simulink library "Driveline_Axle3_A23_A2Diff_A3Diff"  (R2025b)
settings: Solver=VariableStepAuto  StartTime=0.0  StopTime=10.0  RelTol=1e-3
undefined symbols (not defined in the file): Driveline
libraries: Driveshaft_Assembly x4, fl_lib x3, Differential_Systems x2, sdl_lib x2, Driveline_Axle2_A1_A1Diff x2, sm_lib x1
Description:
  | Component of Simscape Vehicle Templates Library
  | 
  | Copyright 2018-2025 The MathWorks, Inc.
settings Model: Creator=smiller  LastModifiedBy=smiller
settings SolverCC: AlgebraicLoopSolver=TrustRegion
settings DataIOCC: ReturnWorkspaceOutputs=off
settings OptimizationCC: ReuseModelBlockBuffer=off
settings DebuggingCC: UnconnectedInputMsg=warning  UnconnectedOutputMsg=warning  UnconnectedLineMsg=warning  ArithmeticOperatorsInVariantConditions=warning
settings ModelReferenceCC: EnableRefExpFcnMdlSchedulingChecks=on
settings SFSimCC: CustomCodeUndefinedFunction=UseInterfaceOnly
settings RTWCC: GPUComputeCapability=3.5  DLArmComputeVersion=19.05

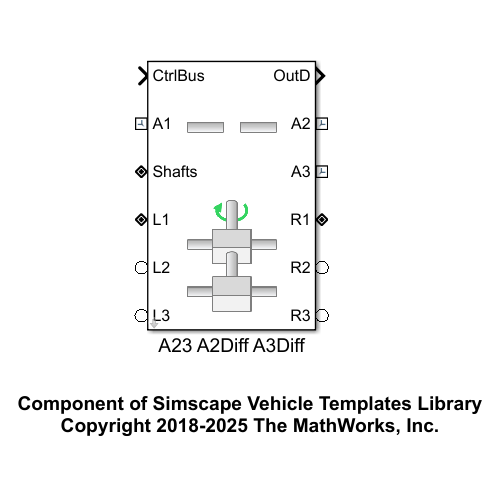
[thumbnail: Simulink's stored preview of the top-level diagram]
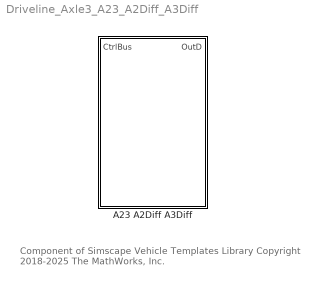
== system Driveline_Axle3_A23_A2Diff_A3Diff ==
  note: Component of Simscape Vehicle Templates Library
      | Copyright 2018-2025 The MathWorks, Inc.
  A23 A2Diff A3Diff : Subsystem  Tag=PublishSubsystem  VariantControl=IndepFRDiffFDiffR  mask(Driveline 6x4, 3-Axle, One Input Shaft){}
      mask help: Models driveline with 3 axles. The second and third axles are mechanically connected, and a single input shaft powers both axles.
      mask Display: image('sm_car_vehicle_driveline_axle3_a23_a2diff_a3diff_IMAGE.png');

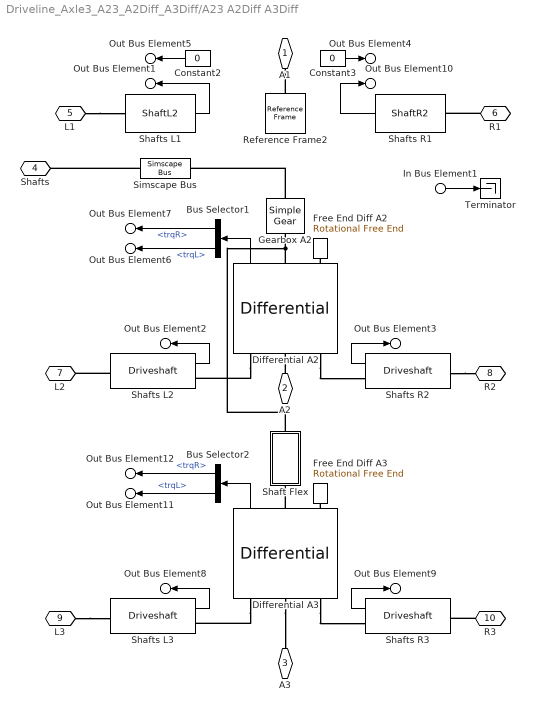
== system Driveline_Axle3_A23_A2Diff_A3Diff/A23 A2Diff A3Diff ==
  In Bus Element1 : Inport  PortName=CtrlBus
  Bus Selector1 : BusSelector  OutputSignals=trqR,trqL
  Bus Selector2 : BusSelector  OutputSignals=trqR,trqL
  Constant2 : Constant  Value=0
  Constant3 : Constant  Value=0
  Differential A2 : Differential_Systems/Differential  VariantControl=Variant1  LabelModeActiveChoice=Gear1DShafts1D  Differential=Driveline.DifferentialA2  VariantLabel=Driveline.DifferentialA2.class.Value
      settings: AttributesFormatString=%<ActiveVariant>
  Differential A3 : Differential_Systems/Differential  VariantControl=Variant1  LabelModeActiveChoice=Gear1DShafts1D  Differential=Driveline.DifferentialA3  VariantLabel=Driveline.DifferentialA3.class.Value
      settings: AttributesFormatString=%<ActiveVariant>
  Free End Diff A2 : fl_lib/Mechanical/Rotational Elements/Rotational Free End  w_specify=off  w_priority=None  w=0 rad/s  w_nominal_specify=off  w_nominal_value=1  w_nominal_unit=rad/s
  Free End Diff A3 : fl_lib/Mechanical/Rotational Elements/Rotational Free End  w_specify=off  w_priority=None  w=0 rad/s  w_nominal_specify=off  w_nominal_value=1  w_nominal_unit=rad/s
  Gearbox A2 : sdl_lib/Gears/Simple Gear  ratio=Driveline.GearboxA2.ratio.Value  rotation_direction=3-2*(1)  friction_model=1  T_noload=0.1 N*m  T_nom=5 N*m  efficiency_nom=0.8  efficiency=0.8  temperature_TLU=[280, 300, 320] K  load_TLU=[1, 5, 10] N*m  efficiency_TLU=[.95, .9, .85]  efficiency_TLU2=[.85, .8, .75; .95, .9, .85; .85, .8, .7]  w_thr=0.01 rad/s  pwr_thr=0.001 W  enable_backlash=false  hardstop_model=simscape.enum.hardstop.smooth  backlash_distance=1e-3 mm  r_base=0.1 m  transition=1e-4 mm  backlash_stiffness=1e7 N/m  backlash_damping=1e6 N*s/m  coeff_rest=0  v_tol=0.001 m/s  f_tol=0 N  mu_visc=[0, 0] N*m/(rad/s)  thermal_mass=50 J/K  temperature_specify=off  temperature_priority=High  temperature=300 K  temperature_nominal_specify=off  temperature_nominal_value=1  temperature_nominal_unit=K  x_backlash_specify=off  x_backlash_priority=None  x_backlash=0 mm  x_backlash_nominal_specify=off  x_backlash_nominal_value=1  x_backlash_nominal_unit=mm  f_hardstop_specify=off  f_hardstop_priority=None  f_hardstop=0 N  f_hardstop_nominal_specify=off  f_hardstop_nominal_value=1  f_hardstop_nominal_unit=N  v_backlash_specify=off  v_backlash_priority=None  v_backlash=0 m/s  v_backlash_nominal_specify=off  v_backlash_nominal_value=1  v_backlash_nominal_unit=m/s
  Reference Frame2 : sm_lib/Frames and Transforms/Reference Frame
  Shaft Flex : Subsystem
  Shafts L1 : Driveline_Axle2_A1_A1Diff/A1 A1Diff/ShaftL2  VariantControl=Shaft1D
  Shafts L2 : Driveshaft_Assembly/Driveshaft  VariantControl=Variant1  LabelModeActiveChoice=Shaft1D  popup_leftRight=Left  Driveshaft=Driveline.DriveshaftL2  VariantLabel=Driveline.DriveshaftL2.class.Value
      settings: AttributesFormatString=%<ActiveVariant>
  Shafts L3 : Driveshaft_Assembly/Driveshaft  VariantControl=Variant1  LabelModeActiveChoice=Shaft1D  popup_leftRight=Left  Driveshaft=Driveline.DriveshaftL3  VariantLabel=Driveline.DriveshaftL3.class.Value
      settings: AttributesFormatString=%<ActiveVariant>
  Shafts R1 : Driveline_Axle2_A1_A1Diff/A1 A1Diff/ShaftR2  VariantControl=Shaft1D
  Shafts R2 : Driveshaft_Assembly/Driveshaft  VariantControl=Variant1  LabelModeActiveChoice=Shaft1D  popup_leftRight=Right  Driveshaft=Driveline.DriveshaftR2  VariantLabel=Driveline.DriveshaftR2.class.Value
      settings: AttributesFormatString=%<ActiveVariant>
  Shafts R3 : Driveshaft_Assembly/Driveshaft  VariantControl=Variant1  LabelModeActiveChoice=Shaft1D  popup_leftRight=Right  Driveshaft=Driveline.DriveshaftR3  VariantLabel=Driveline.DriveshaftR3.class.Value
      settings: AttributesFormatString=%<ActiveVariant>
  Simscape Bus : SimscapeBus  HierarchyStrings=ShaftA2
  Terminator : Terminator
  A1 : PMIOPort  Side=Left
  A2 : PMIOPort  Port=2  Side=Right
  A3 : PMIOPort  Port=3  Side=Right
  Shafts : PMIOPort  Port=4  Side=Left
  L1 : PMIOPort  Port=5  Side=Left
  R1 : PMIOPort  Port=6  Side=Right
  L2 : PMIOPort  Port=7  Side=Left
  R2 : PMIOPort  Port=8  Side=Right
  L3 : PMIOPort  Port=9  Side=Left
  R3 : PMIOPort  Port=10  Side=Right
  Out Bus Element4 : Outport  VectorParamsAs1DForOutWhenUnconnected=off  PortName=OutD  Element=MDriveshaftR1
  Out Bus Element5 : Outport  VectorParamsAs1DForOutWhenUnconnected=off  PortName=OutD  Element=MDriveshaftL1
  Out Bus Element2 : Outport  VectorParamsAs1DForOutWhenUnconnected=off  PortName=OutD  Element=anDriveshaftL2
  Out Bus Element3 : Outport  VectorParamsAs1DForOutWhenUnconnected=off  PortName=OutD  Element=anDriveshaftR2
  Out Bus Element6 : Outport  VectorParamsAs1DForOutWhenUnconnected=off  PortName=OutD  Element=MDriveshaftL2
  Out Bus Element7 : Outport  VectorParamsAs1DForOutWhenUnconnected=off  PortName=OutD  Element=MDriveshaftR2
  Out Bus Element1 : Outport  VectorParamsAs1DForOutWhenUnconnected=off  PortName=OutD  Element=anDriveshaftL1
  Out Bus Element10 : Outport  VectorParamsAs1DForOutWhenUnconnected=off  PortName=OutD  Element=anDriveshaftR1
  Out Bus Element8 : Outport  VectorParamsAs1DForOutWhenUnconnected=off  PortName=OutD  Element=anDriveshaftL3
  Out Bus Element9 : Outport  VectorParamsAs1DForOutWhenUnconnected=off  PortName=OutD  Element=anDriveshaftR3
  Out Bus Element11 : Outport  VectorParamsAs1DForOutWhenUnconnected=off  PortName=OutD  Element=MDriveshaftL3
  Out Bus Element12 : Outport  VectorParamsAs1DForOutWhenUnconnected=off  PortName=OutD  Element=MDriveshaftR3
  wires:
  In Bus Element1/1 -> Terminator/1
  Shafts R2/1 -> Out Bus Element3/1
  Shafts L2/1 -> Out Bus Element2/1
  Differential A2/1 -> Bus Selector1/1
  Bus Selector1/1 -> Out Bus Element7/1  "<trqR>"
  Bus Selector1/2 -> Out Bus Element6/1  "<trqL>"
  Shafts L1/1 -> Out Bus Element1/1
  Shafts R1/1 -> Out Bus Element10/1
  Constant2/1 -> Out Bus Element5/1
  Constant3/1 -> Out Bus Element4/1
  Bus Selector2/2 -> Out Bus Element11/1  "<trqL>"
  Bus Selector2/1 -> Out Bus Element12/1  "<trqR>"
  Differential A3/1 -> Bus Selector2/1
  Shafts L3/1 -> Out Bus Element8/1
  Shafts R3/1 -> Out Bus Element9/1
  connections:
  Simscape Bus/RConn1 -- Shafts/RConn1
  Shafts L2/LConn1 -- L2/RConn1
  Shafts R2/LConn1 -- R2/RConn1
  R3/RConn1 -- Shafts R3/LConn1
  L3/RConn1 -- Shafts L3/LConn1
  A2/RConn1 -- Differential A2/LConn2
  Differential A2/LConn1 -- Shafts L2/RConn1
  Differential A2/LConn3 -- Shafts R2/RConn1
  Gearbox A2/LConn1 -- Simscape Bus/LConn1
  Differential A2/RConn2 -- Free End Diff A2/LConn1
  Differential A2/RConn1 -- Shaft Flex/LConn1 -- Gearbox A2/RConn1
  L1/RConn1 -- Shafts L1/LConn1
  R1/RConn1 -- Shafts R1/LConn1
  Reference Frame2/RConn1 -- A1/RConn1
  Differential A3/RConn2 -- Free End Diff A3/LConn1
  Differential A3/LConn3 -- Shafts R3/RConn1
  Differential A3/LConn1 -- Shafts L3/RConn1
  Differential A3/LConn2 -- A3/RConn1
  Differential A3/RConn1 -- Shaft Flex/RConn1

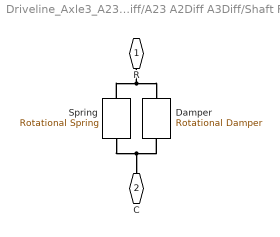
== system Driveline_Axle3_A23_A2Diff_A3Diff/A23 A2Diff A3Diff/Shaft Flex ==
  Damper : sdl_lib/Couplings & Drives/Springs & Dampers/Rotational Damper  D=Driveline.ShaftA23.d.Value N*m/(rad/s)  thermal_port=simscape.enum.thermaleffects.omit  thermal_mass=50 kJ/K  temperature_specify=off  temperature_priority=High  temperature=300 K  temperature_nominal_specify=off  temperature_nominal_value=1  temperature_nominal_unit=K
  Spring : fl_lib/Mechanical/Rotational Elements/Rotational Spring  spr_rate=Driveline.ShaftA23.K.Value N*m/rad  w_specify=off  w_priority=None  w=0 rad/s  w_nominal_specify=off  w_nominal_value=1  w_nominal_unit=rad/s  t_specify=off  t_priority=None  t=0 N*m  t_nominal_specify=off  t_nominal_value=1  t_nominal_unit=N*m  phi_specify=off  phi_priority=High  phi=0 rad  phi_nominal_specify=off  phi_nominal_value=1  phi_nominal_unit=rad
  R : PMIOPort  Side=Left
  C : PMIOPort  Port=2  Side=Right
  connections:
  Spring/RConn1 -- Damper/RConn1 -- C/RConn1
  Spring/LConn1 -- Damper/LConn1 -- R/RConn1
